simulink model "Simulink_buck_model"  (R2020a)
settings: Solver=ode23  StartTime=0.0  StopTime=tsim  FixedStep=1e-6  RelTol=1e-3
values from neighbouring files (symbols this model uses):
  C = 100e-6    (= 0.0001)    [BuckStatespace.m]    (also in Buck_converter_model.m)
  C_p = C    (= 0.0001)    [Buck_converter_model.m]
  D = 0.5    [Buck_converter_model.m]
  fsw = 100e3    (= 100000)    [Buck_converter_model.m]
  i_L_int = 0    [Buck_converter_model.m]
  L = 5e-6    (= 5e-06)    [BuckStatespace.m]    (also in Buck_converter_model.m = 0.0001)
  L_p = L    (= 0.0001)    [Buck_converter_model.m]
  R = 10.0    (= 10)    [BuckStatespace.m]    (also in Buck_converter_model.m)
  r1 = 5e-3    (= 0.005)    [Buck_converter_model.m]
  rc = 5e-3    (= 0.005)    [Buck_converter_model.m]
  rd = 4e-3    (= 0.004)    [Buck_converter_model.m]
  rl = 10e-3    (= 0.01)    [Buck_converter_model.m]
  vd = 0.7    [Buck_converter_model.m]
  Vin = 8    [BuckStatespace.m]    (also in Buck_converter_model.m = 50)
libraries: powerlib x15
settings Model: Creator=mirha  LastModifiedBy=mirha

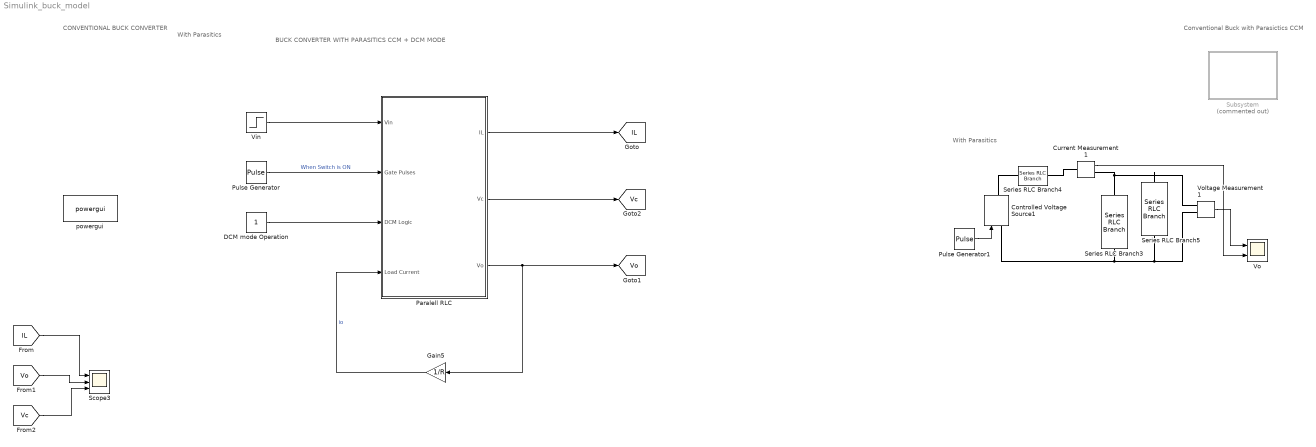
== system Simulink_buck_model ==
  note: BUCK CONVERTER WITH PARASITICS CCM + DCM MODE
  note: Conventional Buck with Parasictics CCM
  note: CONVENTIONAL
      |
      | BUCK CONVERTER
  note: With Parasitics
  note: With Parasitics
  Controlled Voltage Source1 : powerlib/Electrical Sources/Controlled Voltage Source  Initialize=on  Source_Type=AC  Amplitude=0  Phase=0  Frequency=0  Measurements=None
  Current Measurement1 : powerlib/Measurements/Current Measurement  PhasorSimulation=off  OutputType=Complex  PSBequivalent=0
  DCM mode Operation : Constant
  Gain5 : Gain  Gain=1/R
  "Paralell RLC " : Subsystem
  Pulse Generator : DiscretePulseGenerator  PulseType=Time based  Period=1/fsw  PulseWidth=D*100
  Pulse Generator1 : DiscretePulseGenerator  PulseType=Time based  Amplitude=Vin  Period=1e-3  PulseWidth=50
  Scope3 : Scope  NumInputPorts=3
  Series RLC Branch3 : powerlib/Elements/Series RLC Branch  LConnTagsString=__new0  RConnTagsString=__new0  BranchType=R  Resistance=R  Inductance=1e-3  SetiL0=off  InitialCurrent=0  Capacitance=1e-6  Setx0=off  InitialVoltage=0  Measurements=None
  Series RLC Branch4 : powerlib/Elements/Series RLC Branch  LConnTagsString=__new0  RConnTagsString=__new0  BranchType=RL  Resistance=rl  Inductance=L_p  SetiL0=off  InitialCurrent=0  Capacitance=1e-6  Setx0=off  InitialVoltage=0  Measurements=None
  Series RLC Branch5 : powerlib/Elements/Series RLC Branch  LConnTagsString=__new0  RConnTagsString=__new0  BranchType=RC  Resistance=rc  Inductance=L  SetiL0=off  InitialCurrent=0  Capacitance=C_p  Setx0=off  InitialVoltage=0  Measurements=None
  Subsystem : Subsystem  Commented=on
  Vin : Step  Time=7  Before=Vin  After=Vin+5  SampleTime=0
  Vo : Scope  NumInputPorts=2
  Voltage Measurement1 : powerlib/Measurements/Voltage Measurement  PhasorSimulation=off  OutputType=Complex  PSBequivalent=0
  powergui : powerlib/powergui  Priority=1  SimulationMode=Continuous  SampleTime=50e-6  frequency=60  Iterations=50  frequencyindice=0  Pbase=100e6  ErrMax=1e-4  UnitsV=kV  UnitsW=MW  buscounter=0  FunctionMessages=off  echomessages=off  EnableUseOfTLC=off  CurrentSourceSwitches=off  DisableSnubberDevices=off  DisableRonSwitches=off  DisableVfSwitches=off  DisplayEquations=off  AutomaticDiscreteSolvers=off  SolverType=Tustin/Backward Euler (TBE)  Interpol=off  ExternalGateDelay=off  methode=off  Ts=100  x0status=blocks  SPID=on  SwTol=0  HookPort=off  NonlinearTolerance=1e-4  nMaxIteration=100  ContinueOnMaxIteration=off  RestoreLinks=warning  ResistiveCurrentMeasurement=off  Frange=[0:2:500]  Ylog=off  Xlog=on  ShowGrid=off  save=off  variable=ZData  structure=0  ZoomFFT=off  StartTime=0.0  cycles=1  DisplayStyle=1  fundamental=60  FreqAxis=off  MaxFrequency=1000  frequencyindicesteady=1  RmsSteady=1  display=off
  tag scope: IL=global, Vc=global, Vo=global
  wires:
  Current Measurement1/1 -> Vo/2
  Voltage Measurement1/1 -> Vo/1
  Pulse Generator1/1 -> Controlled Voltage Source1/1
  [IL] -> Scope3/1
  [Vo] -> Scope3/2
  [Vc] -> Scope3/3
  "Paralell RLC "/2(Vc) -> [Vc]
  "Paralell RLC "/1(IL) -> [IL]
  Gain5/1 -> "Paralell RLC "/4(Load Current)  "io"
  DCM mode Operation/1 -> "Paralell RLC "/3(DCM Logic)
  Pulse Generator/1 -> "Paralell RLC "/2(Gate Pulses)  "When Switch is ON"
  "Paralell RLC "/3(Vo) -> Gain5/1, [Vo]
  Vin/1 -> "Paralell RLC "/1(Vin)
  connections:
  Series RLC Branch3/LConn1 -- Current Measurement1/RConn1 -- Series RLC Branch5/LConn1 -- Voltage Measurement1/LConn1
  Series RLC Branch3/RConn1 -- Controlled Voltage Source1/LConn1 -- Voltage Measurement1/LConn2 -- Series RLC Branch5/RConn1
  Current Measurement1/LConn1 -- Series RLC Branch4/RConn1
  Controlled Voltage Source1/RConn1 -- Series RLC Branch4/LConn1

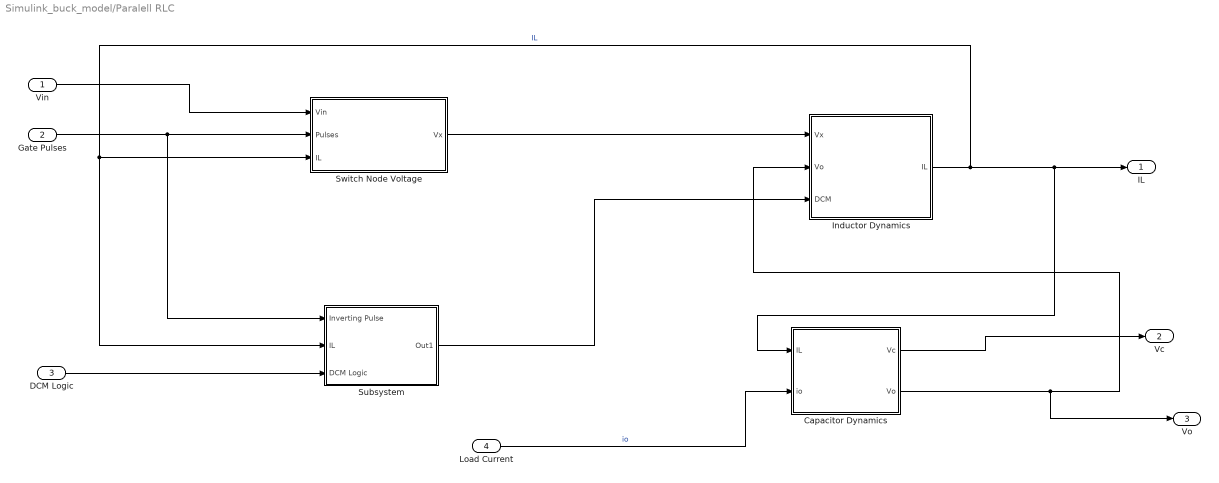
== system Simulink_buck_model/Paralell RLC  ==
  Vin : Inport
  Gate Pulses : Inport  Port=2
  DCM Logic : Inport  Port=3
  Load Current : Inport  Port=4
  Capacitor Dynamics : Subsystem
  Inductor Dynamics : Subsystem
  Subsystem : Subsystem
  Switch Node Voltage : Subsystem
  IL : Outport
  Vc : Outport  Port=2
  Vo : Outport  Port=3
  wires:
  Capacitor Dynamics/2(Vo) -> Vo/1, Inductor Dynamics/2(Vo)
  Load Current/1 -> Capacitor Dynamics/2(io)  "io"
  Switch Node Voltage/1(Vx) -> Inductor Dynamics/1(Vx)
  Inductor Dynamics/1(IL) -> Subsystem/2(IL), Switch Node Voltage/3(IL), IL/1, Capacitor Dynamics/1(IL)  "IL"
  Vin/1 -> Switch Node Voltage/1(Vin)
  Gate Pulses/1 -> Subsystem/1(Inverting Pulse), Switch Node Voltage/2(Pulses)
  DCM Logic/1 -> Subsystem/3(DCM Logic)
  Subsystem/1(Out1) -> Inductor Dynamics/3("DCM ")
  Capacitor Dynamics/1(Vc) -> Vc/1

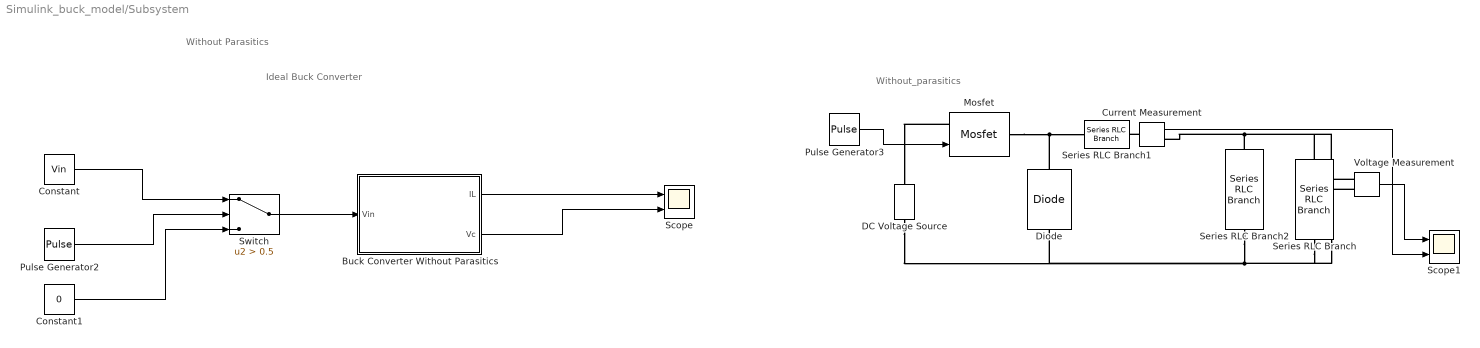
== system Simulink_buck_model/Subsystem ==
  note: Ideal Buck Converter
  note: Without_parasitics
  note: Without Parasitics
  "Buck Converter Without Parasitics " : Subsystem
  Constant : Constant  Value=Vin
  Constant1 : Constant  Value=0
  Current Measurement : powerlib/Measurements/Current Measurement  PhasorSimulation=off  OutputType=Complex  PSBequivalent=0
  DC Voltage Source : powerlib/Electrical Sources/DC Voltage Source  Amplitude=Vin  Measurements=None
  Diode : powerlib/Power Electronics/Diode  Ron=0.001  Lon=0  Vf=0  IC=0  UseSnubber=0  Rs=500  Cs=250e-9  Measurements=off
  Mosfet : powerlib/Power Electronics/Mosfet  Ron=0.1  Lon=0  Rd=0.01  Vfd=0  IC=0  Rs=1e5  Cs=inf  Measurements=off
  Pulse Generator2 : DiscretePulseGenerator  PulseType=Time based  Period=1/100000  PulseWidth=40
  Pulse Generator3 : DiscretePulseGenerator  PulseType=Time based  Period=1/100000  PulseWidth=40
  Scope : Scope  NumInputPorts=2
  Scope1 : Scope  NumInputPorts=2
  Series RLC Branch : powerlib/Elements/Series RLC Branch  LConnTagsString=__new0  RConnTagsString=__new0  BranchType=R  Resistance=R  Inductance=1e-3  SetiL0=off  InitialCurrent=0  Capacitance=1e-6  Setx0=off  InitialVoltage=0  Measurements=None
  Series RLC Branch1 : powerlib/Elements/Series RLC Branch  LConnTagsString=__new0  RConnTagsString=__new0  BranchType=L  Resistance=R  Inductance=L  SetiL0=off  InitialCurrent=0  Capacitance=1e-6  Setx0=off  InitialVoltage=0  Measurements=None
  Series RLC Branch2 : powerlib/Elements/Series RLC Branch  LConnTagsString=__new0  RConnTagsString=__new0  BranchType=C  Resistance=R  Inductance=L  SetiL0=off  InitialCurrent=0  Capacitance=C  Setx0=off  InitialVoltage=0  Measurements=None
  Switch : Switch  Criteria=u2 > Threshold  Threshold=0.5
  Voltage Measurement : powerlib/Measurements/Voltage Measurement  PhasorSimulation=off  OutputType=Complex  PSBequivalent=0
  wires:
  "Buck Converter Without Parasitics "/2(Vc) -> Scope/2
  Current Measurement/1 -> Scope1/2
  Voltage Measurement/1 -> Scope1/1
  Pulse Generator2/1 -> Switch/2
  Constant/1 -> Switch/1
  Constant1/1 -> Switch/3
  Pulse Generator3/1 -> Mosfet/1
  Switch/1 -> "Buck Converter Without Parasitics "/1(Vin)
  "Buck Converter Without Parasitics "/1(IL) -> Scope/1
  connections:
  Series RLC Branch2/RConn1 -- Series RLC Branch/RConn1 -- Voltage Measurement/LConn2 -- DC Voltage Source/LConn1 -- Diode/LConn1
  Series RLC Branch2/LConn1 -- Series RLC Branch/LConn1 -- Voltage Measurement/LConn1 -- Current Measurement/RConn1
  Diode/RConn1 -- Mosfet/RConn1 -- Series RLC Branch1/LConn1
  Mosfet/LConn1 -- DC Voltage Source/RConn1
  Current Measurement/LConn1 -- Series RLC Branch1/RConn1

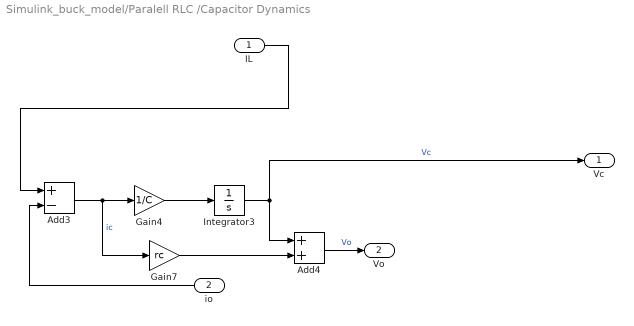
== system Simulink_buck_model/Paralell RLC /Capacitor Dynamics ==
  IL : Inport
  io : Inport  Port=2
  Add3 : Sum  Inputs=+-
  Add4 : Sum
  Gain4 : Gain  Gain=1/C
  Gain7 : Gain  Gain=rc
  Integrator3 : Integrator  InitialCondition=i_L_int
  Vc : Outport
  Vo : Outport  Port=2
  wires:
  Add3/1 -> Gain7/1, Gain4/1  "ic"
  Integrator3/1 -> Vc/1, Add4/1  "Vc"
  Gain4/1 -> Integrator3/1
  Gain7/1 -> Add4/2
  IL/1 -> Add3/1
  io/1 -> Add3/2
  Add4/1 -> Vo/1  "Vo"

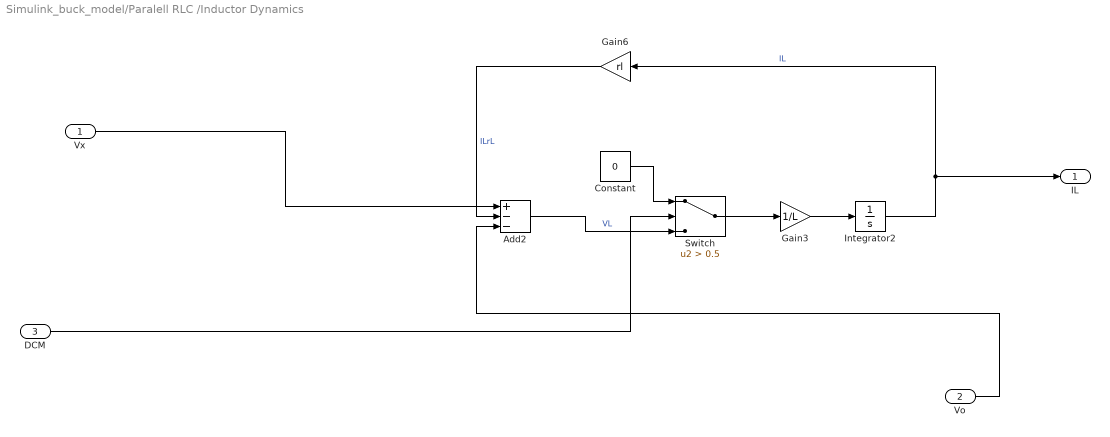
== system Simulink_buck_model/Paralell RLC /Inductor Dynamics ==
  Vx : Inport
  Vo : Inport  Port=2
  "DCM " : Inport  Port=3
  Add2 : Sum  Inputs=+--
  Constant : Constant  Value=0
  Gain3 : Gain  Gain=1/L
  Gain6 : Gain  Gain=rl
  Integrator2 : Integrator  InitialCondition=i_L_int
  Switch : Switch  Criteria=u2 > Threshold  Threshold=0.5
  IL : Outport
  wires:
  Integrator2/1 -> IL/1, Gain6/1  "IL"
  Constant/1 -> Switch/1
  Add2/1 -> Switch/3  "VL"
  Gain3/1 -> Integrator2/1
  Vx/1 -> Add2/1
  Gain6/1 -> Add2/2  "ILrL"
  Switch/1 -> Gain3/1
  Vo/1 -> Add2/3
  "DCM "/1 -> Switch/2

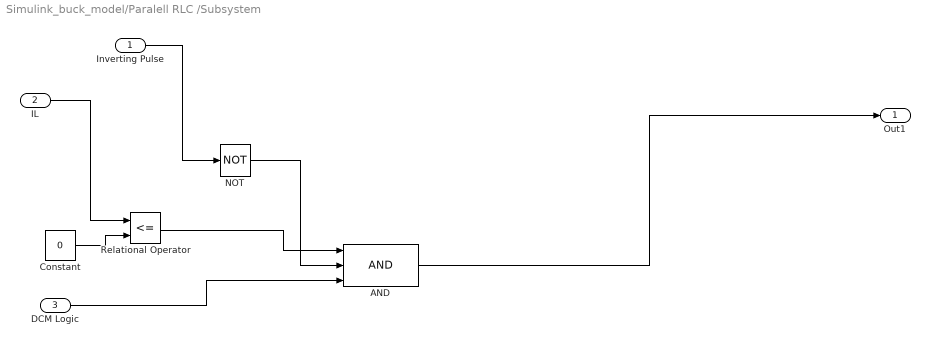
== system Simulink_buck_model/Paralell RLC /Subsystem ==
  Inverting Pulse : Inport
  IL : Inport  Port=2
  DCM Logic : Inport  Port=3
  AND : Logic  Inputs=3  IconShape=distinctive  AllPortsSameDT=off  OutDataTypeStr=boolean
  Constant : Constant  Value=0
  NOT : Logic  Operator=NOT  IconShape=distinctive  AllPortsSameDT=off  OutDataTypeStr=boolean
  Relational Operator : RelationalOperator  Operator=<=  OutDataTypeStr=boolean  RndMeth=Simplest
  Out1 : Outport
  wires:
  Constant/1 -> Relational Operator/2
  IL/1 -> Relational Operator/1
  NOT/1 -> AND/2
  Relational Operator/1 -> AND/1
  DCM Logic/1 -> AND/3
  Inverting Pulse/1 -> NOT/1
  AND/1 -> Out1/1

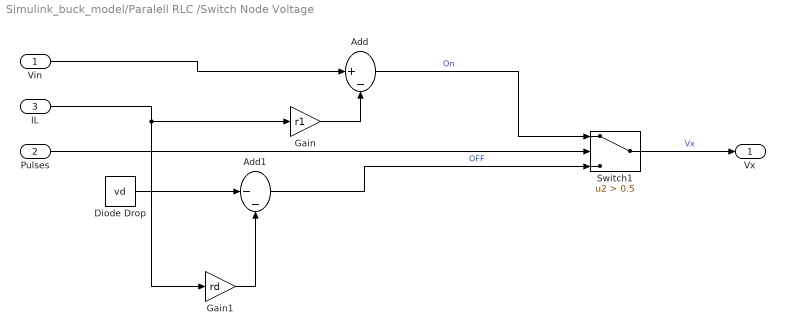
== system Simulink_buck_model/Paralell RLC /Switch Node Voltage ==
  Vin : Inport
  Pulses : Inport  Port=2
  IL : Inport  Port=3
  Add : Sum  Inputs=|+-
  Add1 : Sum  Inputs=|--
  "Diode Drop " : Constant  Value=vd
  Gain : Gain  Gain=r1
  Gain1 : Gain  Gain=rd
  Switch1 : Switch  Criteria=u2 > Threshold  Threshold=0.5
  Vx : Outport
  wires:
  Switch1/1 -> Vx/1  "Vx"
  Vin/1 -> Add/1
  "Diode Drop "/1 -> Add1/1
  IL/1 -> Gain/1, Gain1/1
  Gain1/1 -> Add1/2
  Gain/1 -> Add/2
  Add/1 -> Switch1/1  "On"
  Add1/1 -> Switch1/3  "OFF"
  Pulses/1 -> Switch1/2

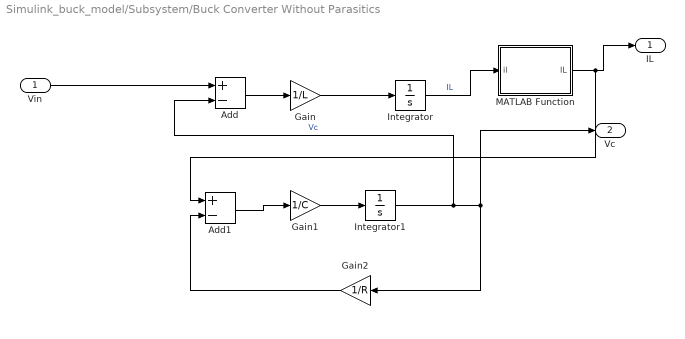
== system Simulink_buck_model/Subsystem/Buck Converter Without Parasitics  ==
  Vin : Inport
  Add : Sum  Inputs=+-
  Add1 : Sum  Inputs=+-
  Gain : Gain  Gain=1/L
  Gain1 : Gain  Gain=1/C
  Gain2 : Gain  Gain=1/R
  Integrator : Integrator  InitialCondition=i_L_int
  Integrator1 : Integrator  InitialCondition=i_L_int
  MATLAB Function : MATLAB Function  TreatAsAtomicUnit=on
  IL : Outport
  Vc : Outport  Port=2
  wires:
  Vin/1 -> Add/1
  Integrator/1 -> MATLAB Function/1(il)  "IL"
  Gain/1 -> Integrator/1
  Gain1/1 -> Integrator1/1
  Gain2/1 -> Add1/2
  Integrator1/1 -> Add/2, Vc/1, Gain2/1  "Vc"
  Add/1 -> Gain/1
  Add1/1 -> Gain1/1
  MATLAB Function/1(IL) -> Add1/1, IL/1

== matlab function Simulink_buck_model/Subsystem/Buck Converter Without Parasitics /MATLAB Function ==
  data: il input; IL output
function IL = fcn(il)

if il <=0
    IL = 0;
else
    IL=il;

end
